simulink model "modelo_linearizacao"  (R2020b)
settings: Solver=VariableStepAuto  StartTime=0.0  StopTime=7  FixedStep=1e-4
undefined symbols (not defined in the file or in its folder): bm1, bm2, bp0, bp1, g, Jm, Jp, kaphi, ku1, ku2, ku3, ku4, l, La, m, Ra
settings Model: Creator=Erick  LastModifiedBy=Erick

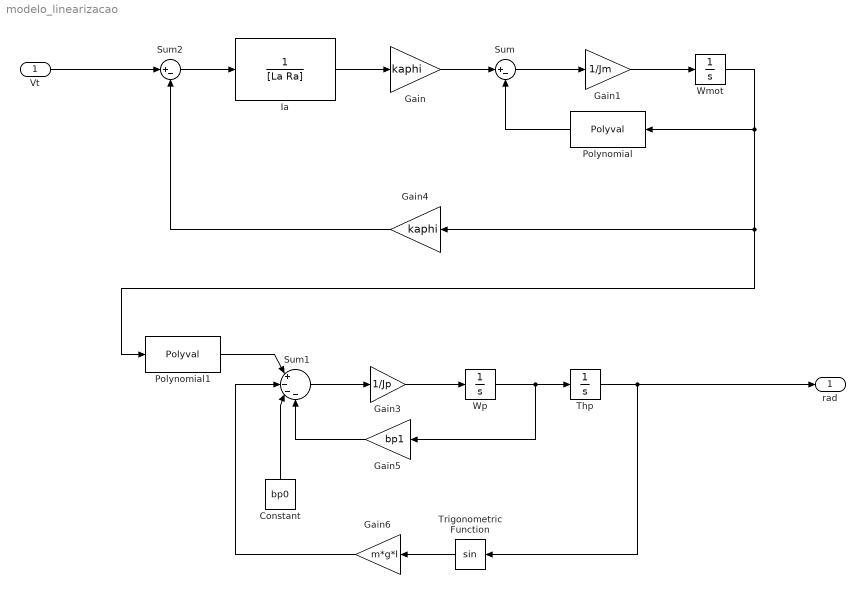
== system modelo_linearizacao ==
  Vt : Inport
  Constant : Constant  Value=bp0
  Gain : Gain  Gain=kaphi
  Gain1 : Gain  Gain=1/Jm
  Gain3 : Gain  Gain=1/Jp
  Gain4 : Gain  Gain=kaphi
  Gain5 : Gain  Gain=bp1
  Gain6 : Gain  Gain=m*g*l
  Ia : TransferFcn  Denominator=[La Ra]
  Polynomial : Polyval  Coefs=[bm2, bm1, 0]
  Polynomial1 : Polyval  Coefs=[ku4, ku3, ku2, ku1, 0]
  Sum : Sum  Inputs=|+-
  Sum1 : Sum  Inputs=|+---
  Sum2 : Sum  Inputs=|+-
  Thp : Integrator  LimitOutput=on  UpperSaturationLimit=deg2rad(90)  LowerSaturationLimit=0
  Trigonometric Function : Trigonometry
  Wmot : Integrator
  Wp : Integrator
  rad : Outport
  wires:
  Constant/1 -> Sum1/3
  Thp/1 -> rad/1, Trigonometric Function/1
  Gain3/1 -> Wp/1
  Polynomial1/1 -> Sum1/1
  Gain6/1 -> Sum1/2
  Wmot/1 -> Polynomial1/1, Gain4/1, Polynomial/1
  Trigonometric Function/1 -> Gain6/1
  Gain1/1 -> Wmot/1
  Sum1/1 -> Gain3/1
  Wp/1 -> Gain5/1, Thp/1
  Vt/1 -> Sum2/1
  Gain/1 -> Sum/1
  Gain5/1 -> Sum1/4
  Sum/1 -> Gain1/1
  Gain4/1 -> Sum2/2
  Sum2/1 -> Ia/1
  Polynomial/1 -> Sum/2
  Ia/1 -> Gain/1
